simulink subsystem "PieroControladoS"  (R2023b)
settings: Solver=VariableStepAuto  StartTime=0.0  StopTime=10.0  RelTol=1e-3
settings Model: Creator=USUARIO  LastModifiedBy=USUARIO

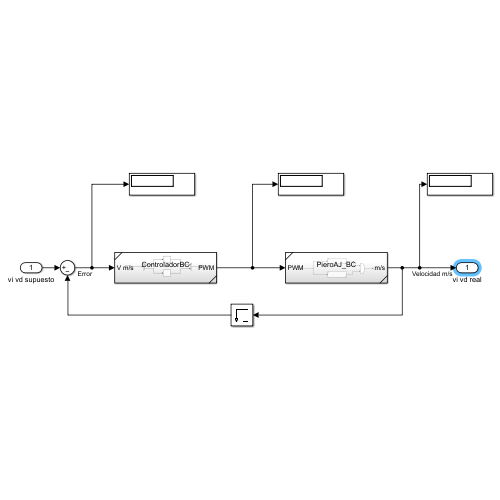
[thumbnail: Simulink's stored preview of the top-level diagram]
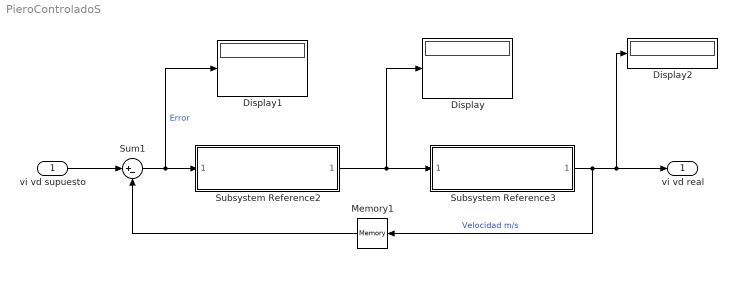
== system PieroControladoS ==
  vi vd supuesto : Inport
  Display : Display
  Display1 : Display
  Display2 : Display
  Memory1 : Memory
  Subsystem Reference2 : Subsystem  ReferencedSubsystem=ControladorBC
  Subsystem Reference3 : Subsystem  ReferencedSubsystem=PieroAJ_BC
  Sum1 : Sum  Inputs=|+-
  vi vd real : Outport
  wires:
  Memory1/1 -> Sum1/2
  Sum1/1 -> Subsystem Reference2/1, Display1/1  "Error"
  Subsystem Reference2/1 -> Subsystem Reference3/1, Display/1
  vi vd supuesto/1 -> Sum1/1
  Subsystem Reference3/1 -> Memory1/1, vi vd real/1, Display2/1  "Velocidad m/s"
